simulink model "Variant_Subsystem"  (R2021b)
settings: Solver=ode4  StartTime=0.0  StopTime=10  FixedStep=0.001  RelTol=1e-3
model workspace (MAT data in the model file):
  Cont_TF_Var = 2
  DE_Var = 4
  Disc_TF_Var = 3
  ODE_Var = 1
  Ts = 0.1
  Variant_Control = 1
  c = 2
  k = 2
  m = 1
settings Model: Creator=amr_y  LastModifiedBy=amr_y

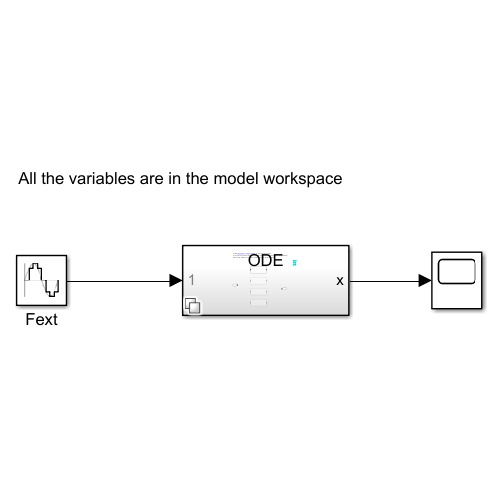
[thumbnail: Simulink's stored preview of the top-level diagram]
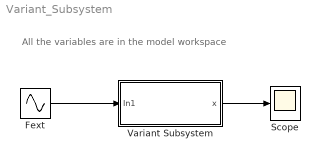
== system Variant_Subsystem ==
  note: All the variables are in the model workspace
  Fext : Sin  SampleTime=Ts
  Scope : Scope
  Variant Subsystem : Subsystem  Variant=on
  wires:
  Fext/1 -> Variant Subsystem/1(In1)
  Variant Subsystem/1(x) -> Scope/1

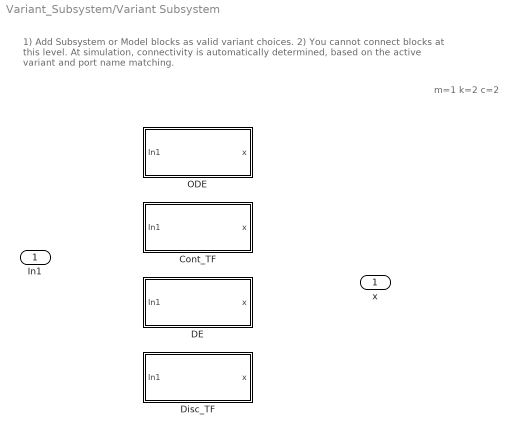
== system Variant_Subsystem/Variant Subsystem ==
  note: 1) Add Subsystem or Model blocks as valid variant choices.
      | 2) You cannot connect blocks at this level. At simulation, connectivity is automatically
      | determined, based on the active variant and port name matching.
  note: m=1
      | k=2
      | c=2
  In1 : Inport
  Cont_TF : Subsystem  VariantControl=Variant_Control==Cont_TF_Var
  DE : Subsystem  VariantControl=Variant_Control==DE_Var
  Disc_TF : Subsystem  VariantControl=Variant_Control==Disc_TF_Var
  ODE : Subsystem  VariantControl=Variant_Control==ODE_Var
  x : Outport

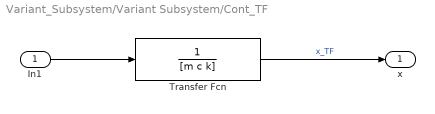
== system Variant_Subsystem/Variant Subsystem/Cont_TF ==
  In1 : Inport
  Transfer Fcn : TransferFcn  Denominator=[m c k]
  x : Outport
  wires:
  Transfer Fcn/1 -> x/1  "x_TF"
  In1/1 -> Transfer Fcn/1

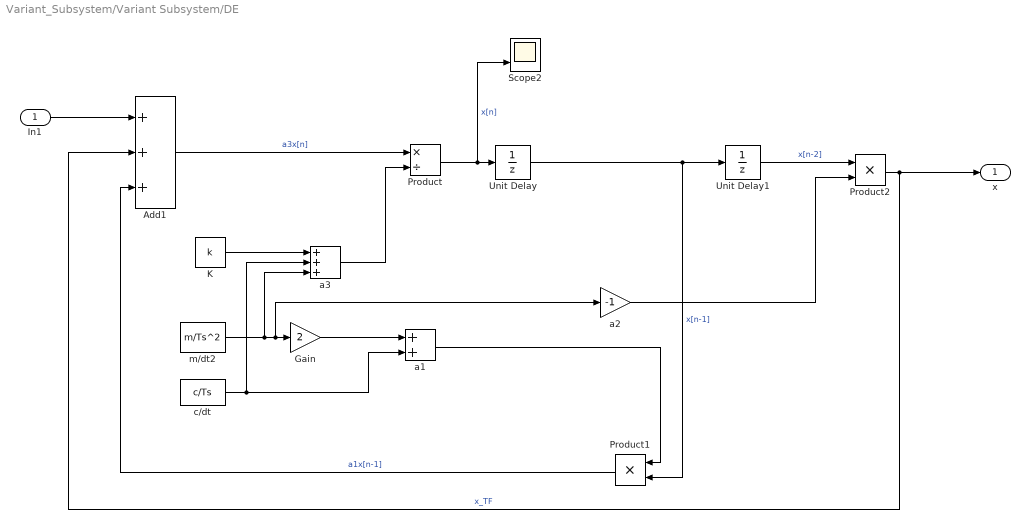
== system Variant_Subsystem/Variant Subsystem/DE ==
  In1 : Inport
  Add1 : Sum  Inputs=+++
  Gain : Gain  Gain=2
  K : Constant  Value=k
  Product : Product  Inputs=*/
  Product1 : Product
  Product2 : Product
  Scope2 : Scope  NumInputPorts=2
  Unit Delay : UnitDelay  SampleTime=-1  HasFrameUpgradeWarning=on
  Unit Delay1 : UnitDelay  SampleTime=-1  HasFrameUpgradeWarning=on
  a1 : Sum
  a2 : Gain  Gain=-1
  a3 : Sum  Inputs=+++
  c/dt : Constant  Value=c/Ts
  m/dt2 : Constant  Value=m/Ts^2
  x : Outport
  wires:
  Product2/1 -> x/1, Add1/2  "x_TF"
  K/1 -> a3/1
  a2/1 -> Product2/2
  Product1/1 -> Add1/3  "a1x[n-1]"
  Unit Delay1/1 -> Product2/1  "x[n-2]"
  Gain/1 -> a1/1
  Unit Delay/1 -> Product1/2, Unit Delay1/1  "x[n-1]"
  a1/1 -> Product1/1
  Add1/1 -> Product/1  "a3x[n]"
  In1/1 -> Add1/1
  Product/1 -> Scope2/2, Unit Delay/1  "x[n]"
  a3/1 -> Product/2
  m/dt2/1 -> a3/3, a2/1, Gain/1
  c/dt/1 -> a3/2, a1/2

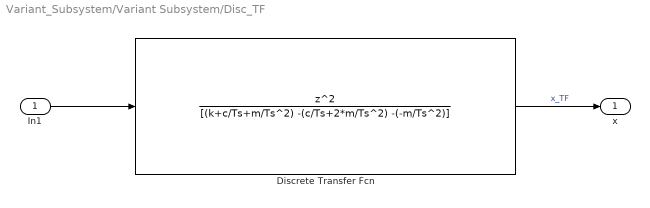
== system Variant_Subsystem/Variant Subsystem/Disc_TF ==
  In1 : Inport
  Discrete Transfer Fcn : DiscreteTransferFcn  Numerator=[1 0 0]  Denominator=[(k+c/Ts+m/Ts^2) -(c/Ts+2*m/Ts^2) -(-m/Ts^2)]  SampleTime=Ts
  x : Outport
  wires:
  Discrete Transfer Fcn/1 -> x/1  "x_TF"
  In1/1 -> Discrete Transfer Fcn/1

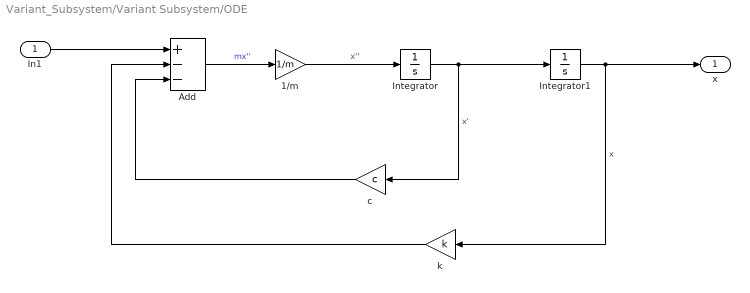
== system Variant_Subsystem/Variant Subsystem/ODE ==
  In1 : Inport
  1/m : Gain  Gain=1/m
  Add : Sum  Inputs=+--
  Integrator : Integrator
  Integrator1 : Integrator
  c : Gain  Gain=c
  k : Gain  Gain=k
  x : Outport
  wires:
  k/1 -> Add/2
  c/1 -> Add/3
  In1/1 -> Add/1
  Add/1 -> 1/m/1  "mx''"
  1/m/1 -> Integrator/1  "x''"
  Integrator1/1 -> x/1, k/1  "x"
  Integrator/1 -> c/1, Integrator1/1  "x'"
